simulink model "CLIK_secondo_ordine"  (R2022b)
settings: Solver=VariableStepAuto  StartTime=0.0  StopTime=40  RelTol=1e-3
values from neighbouring files (symbols this model uses):
  k_d = 20    [CLIK_script.m]
  k_p = (k_d^2)/2    (= 200)    [CLIK_script.m]
  T = T_A * T_B    [DH_dinamica.m]    (also in traiettoria_script.m = 0.001)
  theta1_0 = pi/2 - angolo    [CLIK_script.m]
  theta2_0 = 2*angolo    [CLIK_script.m]
undefined symbols (not defined in the file or in its folder): DiscIntNeverNeededParam
settings Model: Creator=Michele  LastModifiedBy=Michele
settings DataIOCC: ReturnWorkspaceOutputs=off

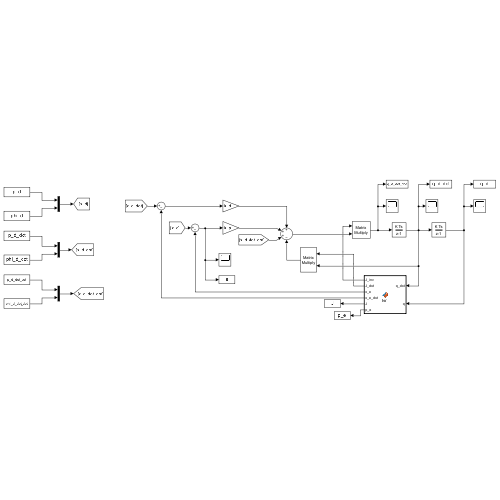
[thumbnail: Simulink's stored preview of the top-level diagram]
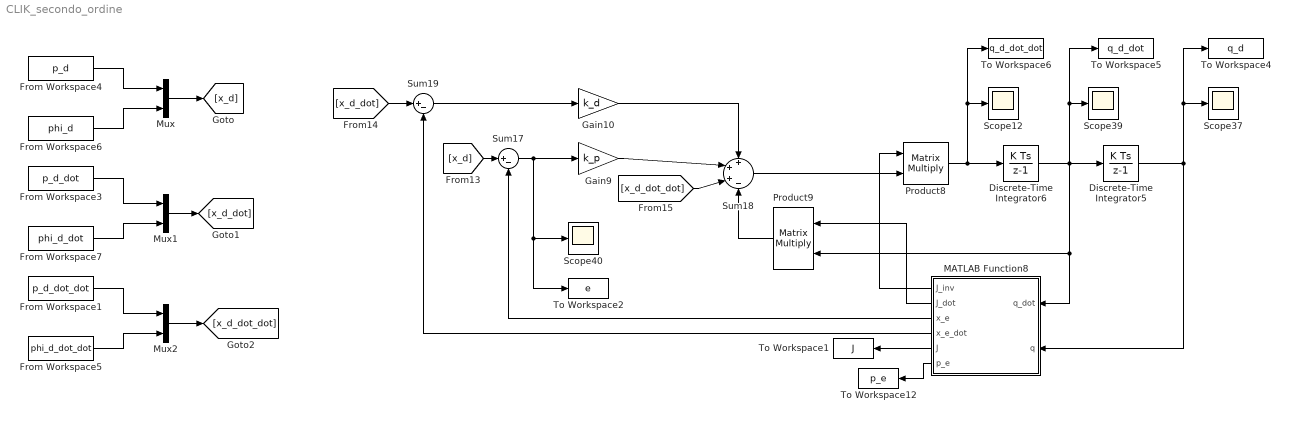
== system CLIK_secondo_ordine ==
  Discrete-Time Integrator5 : DiscreteIntegrator  InitialCondition=[theta1_0 theta2_0 -0.25 0]'  SampleTime=-1  ICPrevOutput=DiscIntNeverNeededParam  ICPrevScaledInput=DiscIntNeverNeededParam
  Discrete-Time Integrator6 : DiscreteIntegrator  InitialCondition=[0 0 0 0]'  SampleTime=-1  ICPrevOutput=DiscIntNeverNeededParam  ICPrevScaledInput=DiscIntNeverNeededParam
  From Workspace1 : FromWorkspace  VariableName=p_d_dot_dot  SampleTime=T
  From Workspace3 : FromWorkspace  VariableName=p_d_dot  SampleTime=T
  From Workspace4 : FromWorkspace  VariableName=p_d  SampleTime=T
  From Workspace5 : FromWorkspace  VariableName=phi_d_dot_dot  SampleTime=T
  From Workspace6 : FromWorkspace  VariableName=phi_d  SampleTime=T
  From Workspace7 : FromWorkspace  VariableName=phi_d_dot  SampleTime=T
  Gain10 : Gain  Gain=k_d
  Gain9 : Gain  Gain=k_p
  MATLAB Function8 : MATLAB Function  TreatAsAtomicUnit=on
  Mux : Mux  Inputs=2
  Mux1 : Mux  Inputs=2
  Mux2 : Mux  Inputs=2
  Product8 : Product  Multiplication=Matrix(*)
  Product9 : Product  Multiplication=Matrix(*)
  Scope{12,37,39..40} (4 alike) : Scope
  Sum17 : Sum  Inputs=|+-
  Sum18 : Sum  Inputs=+++-
  Sum19 : Sum  Inputs=|+-
  To Workspace1 : ToWorkspace  VariableName=J  SaveFormat=Structure With Time  SampleTime=-1
  To Workspace12 : ToWorkspace  VariableName=p_e  SaveFormat=Structure With Time  SampleTime=-1
  To Workspace2 : ToWorkspace  VariableName=e  SaveFormat=Structure With Time  SampleTime=-1
  To Workspace4 : ToWorkspace  VariableName=q_d  SaveFormat=Structure With Time  SampleTime=-1
  To Workspace5 : ToWorkspace  VariableName=q_d_dot  SaveFormat=Structure With Time  SampleTime=-1
  To Workspace6 : ToWorkspace  VariableName=q_d_dot_dot  SaveFormat=Structure With Time  SampleTime=-1
  wires:
  From Workspace4/1 -> Mux/1
  From Workspace6/1 -> Mux/2
  From Workspace3/1 -> Mux1/1
  From Workspace7/1 -> Mux1/2
  From Workspace5/1 -> Mux2/2
  From Workspace1/1 -> Mux2/1
  Mux/1 -> [x_d]
  Mux1/1 -> [x_d_dot]
  Mux2/1 -> [x_d_dot_dot]
  Discrete-Time Integrator6/1 -> To Workspace5/1, Scope39/1, Discrete-Time Integrator5/1, Product9/2, MATLAB Function8/1(q_dot)
  MATLAB Function8/3(x_e) -> Sum17/2
  Sum18/1 -> Product8/2
  MATLAB Function8/2(J_dot) -> Product9/1
  Product8/1 -> Discrete-Time Integrator6/1, To Workspace6/1, Scope12/1
  Discrete-Time Integrator5/1 -> To Workspace4/1, Scope37/1, MATLAB Function8/2(q)
  Gain9/1 -> Sum18/2
  [x_d] -> Sum17/1
  Gain10/1 -> Sum18/1
  MATLAB Function8/4(x_e_dot) -> Sum19/2
  [x_d_dot] -> Sum19/1
  Sum17/1 -> To Workspace2/1, Scope40/1, Gain9/1
  Sum19/1 -> Gain10/1
  [x_d_dot_dot] -> Sum18/3
  Product9/1 -> Sum18/4
  MATLAB Function8/1(J_inv) -> Product8/1
  MATLAB Function8/5(J) -> To Workspace1/1
  MATLAB Function8/6(p_e) -> To Workspace12/1

== matlab function CLIK_secondo_ordine/MATLAB Function8 ==
  data: J_inv output; J_dot output; x_e output; x_e_dot output; q_dot input; q input; J output; p_e output
function [J_inv,J_dot,x_e,x_e_dot,J,p_e] = kin(q_dot,q)

    q1 = q(1); q2 = q(2); q3 = q(3); q4 = q(4);
    q_dot1 = q_dot(1); q_dot2 = q_dot(2); q_dot3 = q_dot(3); q_dot4 = q_dot(4);

    J = [- sin(q1)/2 - (cos(q1)*sin(q2))/2 - (cos(q2)*sin(q1))/2, - (cos(q1)*sin(q2))/2 - (cos(q2)*sin(q1))/2, 0, 0;
           cos(q1)/2 + (cos(q1)*cos(q2))/2 - (sin(q1)*sin(q2))/2,   (cos(q1)*cos(q2))/2 - (sin(q1)*sin(q2))/2, 0, 0;
                                                               0,                                           0, 1, 0;
                                                               0,                                           0, 0, 1];

    x_e = [cos(q1)/2 + (cos(q1)*cos(q2))/2 - (sin(q1)*sin(q2))/2;
           sin(q1)/2 + (cos(q1)*sin(q2))/2 + (cos(q2)*sin(q1))/2;
                                                   q3;
                                                   q4];
    
    J_inv = inv(J);

    J_dot = [- q_dot2*((cos(q1)*cos(q2))/2 - (sin(q1)*sin(q2))/2) - q_dot1*(cos(q1)/2 + (cos(q1)*cos(q2))/2 - (sin(q1)*sin(q2))/2), (q_dot1*cos(q1))/2 - q_dot1*(cos(q1)/2 + (cos(q1)*cos(q2))/2 - (sin(q1)*sin(q2))/2) - q_dot2*((cos(q1)*cos(q2))/2 - (sin(q1)*sin(q2))/2), 0, 0;
             - q_dot2*((cos(q1)*sin(q2))/2 + (cos(q2)*sin(q1))/2) - q_dot1*(sin(q1)/2 + (cos(q1)*sin(q2))/2 + (cos(q2)*sin(q1))/2), (q_dot1*sin(q1))/2 - q_dot1*(sin(q1)/2 + (cos(q1)*sin(q2))/2 + (cos(q2)*sin(q1))/2) - q_dot2*((cos(q1)*sin(q2))/2 + (cos(q2)*sin(q1))/2), 0, 0;
                                                                                                                                 0,                                                                                                                                        0, 0, 0;
                                                                                                                                 0,                                                                                                                                        0, 0, 0];

    x_e_dot = J*q_dot;

    p_e = x_e(1:3);
end
